simulink model "lab5_v1"  (R2015a)
settings: Solver=FixedStepDiscrete  StartTime=0.0  StopTime=1000  FixedStep=1  RelTol=1e-3
libraries: simulink x1
settings Model: CovModelRefEnable=off  Creator=michael  LastModifiedBy=Bruno
settings DataIOCC: SaveFormat=Dataset
settings HardwareCC: ProdBitPerPointer=64  ProdLargestAtomicFloat=Float  ProdIntDivRoundTo=Zero  ProdEndianess=LittleEndian  ProdHWDeviceType=Specified
settings GRTTargetCC: GeneratePreprocessorConditionals=Use local settings

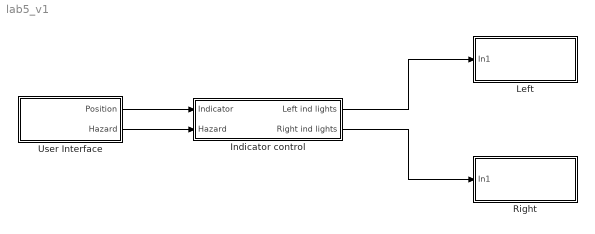
== system lab5_v1 ==
  Indicator control : Subsystem
  Left : Subsystem
  Right : Subsystem
  User Interface : Subsystem
  wires:
  User Interface/1(Position) -> Indicator control/1(Indicator)
  Indicator control/1(Left ind lights) -> Left/1(In1)
  Indicator control/2(Right ind lights) -> Right/1(In1)
  User Interface/2(Hazard) -> Indicator control/2(Hazard)

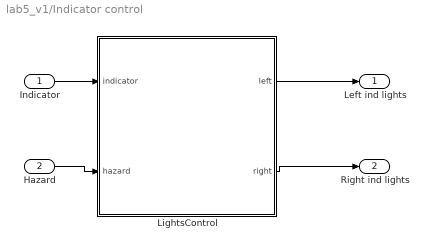
== system lab5_v1/Indicator control ==
  Indicator : Inport
  Hazard : Inport  Port=2
  LightsControl : Stateflow chart  TreatAsAtomicUnit=on
  Left ind lights : Outport
  Right ind lights : Outport  Port=2
  wires:
  Indicator/1 -> LightsControl/1(indicator)
  LightsControl/1(left) -> Left ind lights/1
  LightsControl/2(right) -> Right ind lights/1
  Hazard/1 -> LightsControl/2(hazard)

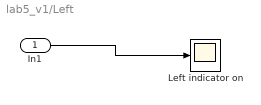
== system lab5_v1/Left ==
  In1 : Inport
  Left indicator on : Scope
      settings: YMin=-0.125  YMax=1.125
  wires:
  In1/1 -> Left indicator on/1

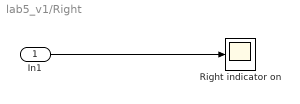
== system lab5_v1/Right ==
  In1 : Inport
  Right indicator on : Scope
      settings: YMin=-0.125  YMax=1.125
  wires:
  In1/1 -> Right indicator on/1

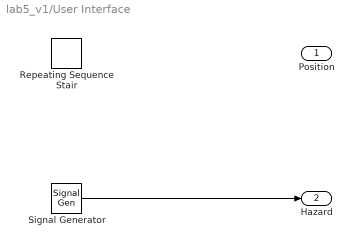
== system lab5_v1/User Interface ==
  Repeating Sequence Stair : simulink/Sources/Repeating Sequence Stair  OutValues=[0 0 -1 -1 1 0 -1 1].'  tsamp=-1  OutMin=[]  OutMax=[]  OutDataTypeStr=double  OutputDataTypeScalingMode=double  OutDataType=fixdt(0,8)  ConRadixGroup=Best Precision: Vector-wise  OutScaling=2^-12
  Signal Generator : SignalGenerator  WaveForm=square
  Position : Outport
  Hazard : Outport  Port=2
  wires:
  ? -> Position/1
  Signal Generator/1 -> Hazard/1

== stateflow chart lab5_v1/Indicator control/LightsControl ==
  state Left
    entry:
  state delay(time) [function]
    (junction 54) -> (junction 55) [order 1] : [i<time]
    (default) -> (junction 55) : {i=0}
    (junction 55) -> (junction 54) : {i = i + 1}
    (junction 54) -> (junction 56) [order 2]
  state Off
    entry:
    left=0; right=0
  state Right
    entry:
  state LeftIndicator
    state Off
      entry:
      right=0; left=0
      during: delay(10)
    state On
      entry:
      right=0; left=1
      during: delay(10)
    LeftIndicator.On -> LeftIndicator.Off
    (default) -> LeftIndicator.Off
    LeftIndicator.Off -> LeftIndicator.On
  state HazardOn
    entry:
  state RightIndicator
    state Off
      entry:
      right=0; left=0
      during: delay(10)
    state On
      entry:
      right=1; left=0
      during: delay(10)
    RightIndicator.On -> RightIndicator.Off
    (default) -> RightIndicator.Off
    RightIndicator.Off -> RightIndicator.On
  Right -> Left [order 2] : [indicator==1;]
  Left -> Right [order 1] : [indicator==-1]
  Off -> Left [order 1] : [indicator==1]
  Left -> Off [order 2] : [indicator==0]
  Off -> Right [order 3] : [indicator==-1]
  (default) -> Off
  Right -> Off [order 1] : [indicator==0]
  HazardOn -> Off : [~hazard]
  Off -> HazardOn [order 2] : [hazard]
  data: time function_input; indicator input; left output; right output; hazard input; i local
